simulink library "MBDS_Applications"  (R2018b)
settings: Solver=ode45  StartTime=0.0  StopTime=10.0  RelTol=1e-3
undefined symbols (not defined in the file or in its folder): Ts
libraries: KIBES_Signal x297, simulink x7
(part 1 of 6)
Description:
  | MBDS project library for Application models
settings Model: Creator=uid60719  LastModifiedBy=uidf0608
settings DataIOCC: LimitDataPoints=on  SaveFormat=Array  SignalLoggingSaveFormat=ModelDataLogs
settings OptimizationCC: BlockReduction=off  BooleanDataType=off  ExpressionDepthLimit=2147483647  LifeSpan=inf
settings DebuggingCC: SaveWithParameterizedLinksMsg=none  UnderspecifiedInitializationDetection=Classic  MergeDetectMultiDrivingBlocksExec=none  SignalResolutionControl=TryResolveAllWithWarning  MultiTaskCondExecSysMsg=none  FcnCallInpInsideContextMsg=warning  AllowSymbolicDim=off  StateNameClashWarn=warning  SFUnexpectedBacktrackingDiag=warning  SFNoUnconditionalDefaultTransitionDiag=warning  SFExecutionAtInitializationDiag=none
settings HardwareCC: ProdBitPerPointer=32  ProdBitPerSizeT=32  ProdBitPerPtrDiffT=32  ProdLargestAtomicFloat=None  ProdIntDivRoundTo=Undefined  ProdEndianess=Unspecified  ProdWordSize=32  ProdHWDeviceType=32-bit Generic  TargetUnknown=on
settings ModelReferenceCC: PropagateSignalLabelsOutOfModel=off
settings SFSimCC: SimUseLocalCustomCode=off
settings RTWCC: RTWUseLocalCustomCode=off
settings CodeAppCC: StateflowObjectComments=on
settings GRTTargetCC: TargetLangStandard=C89/C90 (ANSI)  GeneratePreprocessorConditionals=Disable all  CombineOutputUpdateFcns=off  GRTInterface=on
settings ConfigComp: CovMetricSettings=dw  CovHtmlReporting=on  CovSaveCumulativeToWorkspaceVar=on  CovSaveSingleToWorkspaceVar=on  CovExternalEMLEnable=off  CovSFcnEnable=off

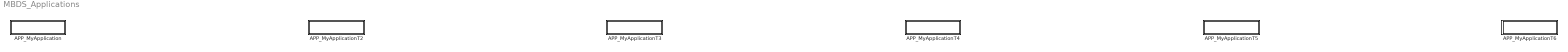
== system MBDS_Applications ==
  APP_MyApplication : Subsystem  mask(APP_MyApplication){MBDS_ElementType=Application, MBDS_WorkStatus=In Work, MBDS_LastModified=2021-02-03-13:46:18}
      mask prompts: MBDS_ElementType "MBDS element type:"; MBDS_WorkStatus "Work status:"; MBDS_LastModified "Last modified:"
      mask help: MBDS Application APP_MyApplication
      settings: CopyFcn=|
      | if(~strcmpi(GetElementType(bdroot(gcs)), 'System'))
      | RemoveBlockMsg(gcb, 'Application blocks can be used in system design models only. The added block instance will be removed from your model to avoid errors.');
      | end
      mask Help: eval(['open([workdir(''help_dir:''),''\MBDS_ProjectLibrary.html''])'])
      mask Display: disp('V 1.115')
  APP_MyApplicationT2 : Subsystem  Description=MyApplicationT2  mask(APP_MyApplicationT2){MBDS_ElementType=Application, MBDS_WorkStatus=In Work, MBDS_LastModified=2021-02-03-13:46:32}
      mask prompts: MBDS_ElementType "MBDS element type:"; MBDS_WorkStatus "Work status:"; MBDS_LastModified "Last modified:"
      mask help: MyApplicationT2
      settings: CopyFcn=|
      | if(~strcmpi(GetElementType(bdroot(gcs)), 'System'))
      | RemoveBlockMsg(gcb, 'Application blocks can be used in system design models only. The added block instance will be removed from your model to avoid errors.');
      | end
      mask Help: eval(['open([workdir(''help_dir:''),''\MBDS_ProjectLibrary.html''])'])
      mask Display: disp('V 1.5')
  APP_MyApplicationT3 : Subsystem  Description=MyApplicationT3  mask(APP_MyApplicationT3){MBDS_ElementType=Application, MBDS_WorkStatus=In Work, MBDS_LastModified=2021-02-03-13:46:39}
      mask prompts: MBDS_ElementType "MBDS element type:"; MBDS_WorkStatus "Work status:"; MBDS_LastModified "Last modified:"
      mask help: MyApplicationT3
      settings: CopyFcn=|
      | if(~strcmpi(GetElementType(bdroot(gcs)), 'System'))
      | RemoveBlockMsg(gcb, 'Application blocks can be used in system design models only. The added block instance will be removed from your model to avoid errors.');
      | end
      mask Help: eval(['open([workdir(''help_dir:''),''\MBDS_ProjectLibrary.html''])'])
      mask Display: disp('V 1.3')
  APP_MyApplicationT4 : Subsystem  Description=MyApplicationT4  mask(APP_MyApplicationT4){MBDS_ElementType=Application, MBDS_WorkStatus=In Work, MBDS_LastModified=2021-02-03-13:46:48}
      mask prompts: MBDS_ElementType "MBDS element type:"; MBDS_WorkStatus "Work status:"; MBDS_LastModified "Last modified:"
      mask help: MyApplicationT4
      settings: CopyFcn=|
      | if(~strcmpi(GetElementType(bdroot(gcs)), 'System'))
      | RemoveBlockMsg(gcb, 'Application blocks can be used in system design models only. The added block instance will be removed from your model to avoid errors.');
      | end
      mask Help: eval(['open([workdir(''help_dir:''),''\MBDS_ProjectLibrary.html''])'])
      mask Display: disp('V 1.11')
  APP_MyApplicationT5 : Subsystem  Description=MyApplicationT5  mask(APP_MyApplicationT5){MBDS_ElementType=Application, MBDS_WorkStatus=In Work, MBDS_LastModified=2021-02-03-13:46:56}
      mask prompts: MBDS_ElementType "MBDS element type:"; MBDS_WorkStatus "Work status:"; MBDS_LastModified "Last modified:"
      mask help: MyApplicationT5
      settings: CopyFcn=|
      | if(~strcmpi(GetElementType(bdroot(gcs)), 'System'))
      | RemoveBlockMsg(gcb, 'Application blocks can be used in system design models only. The added block instance will be removed from your model to avoid errors.');
      | end
      mask Help: eval(['open([workdir(''help_dir:''),''\MBDS_ProjectLibrary.html''])'])
      mask Display: disp('V 1.9')
  APP_MyApplicationT6 : Subsystem  Description=MyApplicationT6  mask(APP_MyApplicationT6){MBDS_ElementType=Application, MBDS_WorkStatus=In Work, MBDS_LastModified=2021-02-03-13:47:04}
      mask prompts: MBDS_ElementType "MBDS element type:"; MBDS_WorkStatus "Work status:"; MBDS_LastModified "Last modified:"
      mask help: MyApplicationT6
      settings: CopyFcn=|
      | if(~strcmpi(GetElementType(bdroot(gcs)), 'System'))
      | RemoveBlockMsg(gcb, 'Application blocks can be used in system design models only. The added block instance will be removed from your model to avoid errors.');
      | end
      mask Help: eval(['open([workdir(''help_dir:''),''\MBDS_ProjectLibrary.html''])'])
      mask Display: disp('V 1.5')

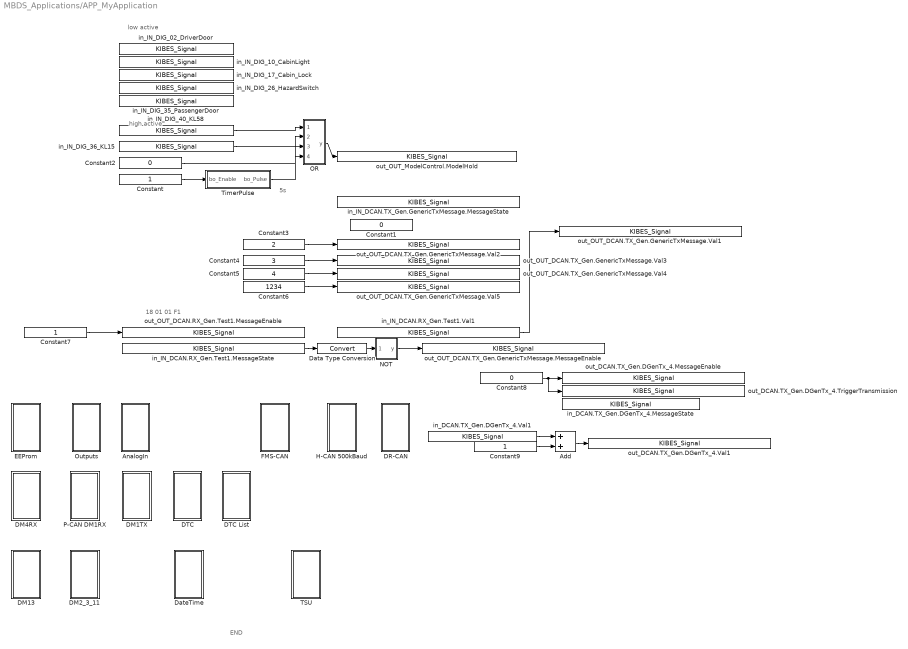
== system MBDS_Applications/APP_MyApplication ==
  note: low active
  note: 5s
  note: high active
  note: 18 01 01 F1
  note: END
  Add : Sum  InitFcn=|  OutDataTypeStr=Inherit: Inherit via back propagation  SaturateOnIntegerOverflow=on
      | if(exist('MBDS_BlockCallback', 'file'))
      |    MBDS_BlockCallback('Update', gcb);  
      | end
      settings: AttributesFormatString=Saturate: %<SaturateOnIntegerOverflow>
  AnalogIn : Subsystem
  Constant : Constant  InitFcn=|  OutDataTypeStr=boolean
      | if(exist('MBDS_BlockCallback', 'file'))
      |    MBDS_BlockCallback('Update', gcb);  
      | end
  Constant1 : Constant  InitFcn=|  Value=0  OutDataTypeStr=boolean
      | if(exist('MBDS_BlockCallback', 'file'))
      |    MBDS_BlockCallback('Update', gcb);  
      | end
  Constant2 : Constant  InitFcn=|  Value=0  OutDataTypeStr=boolean
      | if(exist('MBDS_BlockCallback', 'file'))
      |    MBDS_BlockCallback('Update', gcb);  
      | end
  Constant3 : Constant  InitFcn=|  Value=2  OutDataTypeStr=uint8
      | if(exist('MBDS_BlockCallback', 'file'))
      |    MBDS_BlockCallback('Update', gcb);  
      | end
  Constant4 : Constant  InitFcn=|  Value=3  OutDataTypeStr=uint8
      | if(exist('MBDS_BlockCallback', 'file'))
      |    MBDS_BlockCallback('Update', gcb);  
      | end
  Constant5 : Constant  InitFcn=|  Value=4  OutDataTypeStr=uint8
      | if(exist('MBDS_BlockCallback', 'file'))
      |    MBDS_BlockCallback('Update', gcb);  
      | end
  Constant6 : Constant  InitFcn=|  Value=1234  OutDataTypeStr=uint32
      | if(exist('MBDS_BlockCallback', 'file'))
      |    MBDS_BlockCallback('Update', gcb);  
      | end
  Constant7 : Constant  InitFcn=|  OutDataTypeStr=boolean
      | if(exist('MBDS_BlockCallback', 'file'))
      |    MBDS_BlockCallback('Update', gcb);  
      | end
  Constant8 : Constant  InitFcn=|  Value=0  OutDataTypeStr=boolean
      | if(exist('MBDS_BlockCallback', 'file'))
      |    MBDS_BlockCallback('Update', gcb);  
      | end
  Constant9 : Constant  InitFcn=|  OutDataTypeStr=uint32
      | if(exist('MBDS_BlockCallback', 'file'))
      |    MBDS_BlockCallback('Update', gcb);  
      | end
  DM13 : Subsystem
  DM1TX : Subsystem
  DM2_3_11 : Subsystem
  DM4RX : Subsystem
  DR-CAN : Subsystem
  DTC : Subsystem
  DTC List : Subsystem
  Data Type Conversion : DataTypeConversion  InitFcn=|  SaturateOnIntegerOverflow=on
      | try
      |    MBDS_BlockCallback('Update', gcb);
      | end
      settings: AttributesFormatString=Saturate: %<SaturateOnIntegerOverflow>
  DateTime : Subsystem
  EEProm : Subsystem
  FMS-CAN : Subsystem
  H-CAN 500kBaud : Subsystem
  NOT : Subsystem  InitFcn=|  mask(NOT){MBDS_LibraryBlock=on, BitwiseMode=off, Inputs=1, UseBitMask=off, BitMask='A1', OutDataTypeStr=Inherit: Inherit via back propagation, MBDS_BlockVersion=07.21.05}
      | if(exist('MBDS_BlockCallback', 'file'))
      |    MBDS_BlockCallback('Update', gcb);
      | end
      mask prompts: MBDS_LibraryBlock "MBDS library block"; BitwiseMode "Use 'bitwise' mode"; Inputs "Number of input ports:"; UseBitMask "Use bit mask"; BitMask "Bit mask:"; OutDataTypeStr "Output data type:"; MBDS_BlockVersion "Version:"
      mask help: Logical or bitwise NOT operator. The input value is inverted. In bitwise mode all bits of the input signal are inverted.
      mask init:
      | if(exist('MBDS_BlockCallback', 'file'))
      |    MBDS_BlockCallback('Init', gcb);
      | else
      |    % Disable all mask parameters
      |    MaskEnables = get_param(gcb, 'MaskEnables');
      |    for k = [1:length(MaskEnables)]
      |       MaskEnables{k} = 'off';
      |    end
      |    if(~isequal(MaskEnables, get_param(gcb, 'MaskEnables')))
      |       set_param(gcb, 'MaskEnables', MaskEnables);
      |    end
      | end
      mask Help: eval(['open([workdir(''library_dir:''),''\Blockset\help\'',get_param(gcb,''MaskType''),''.html''])'])
      mask Callback BitwiseMode:
      | if(exist('MBDS_BlockCallback', 'file'))
      |    MBDS_BlockCallback('BitwiseMode', gcb);
      | end
      mask TypeOptions OutDataTypeStr: Inherit: Inherit via back propagation | int8 | uint8 | int16 | uint16 | int32 | uint32 | boolean
      mask Callback OutDataTypeStr:
      | % Adopt Value
      | if(exist('MBDS_BlockCallback', 'file'))
      |    MBDS_BlockCallback('OutDataTypeStr', gcb);
      | end
      mask DialogControl ParameterTabVar0 Prompt: Main
      mask DialogControl ParameterTabVar01 Prompt: Signal Attributes
      mask DialogControl ParameterTabVar012 Prompt: Version
      mask Display:
      | % Show icon or block text
      | disp('NOT')
  OR : Subsystem  InitFcn=|  mask(OR){MBDS_LibraryBlock=on, BitwiseMode=off, Inputs=4, UseBitMask=off, BitMask='A1', OutDataTypeStr=Inherit: Inherit via back propagation, MBDS_BlockVersion=07.21.05}
      | if(exist('MBDS_BlockCallback', 'file'))
      |    MBDS_BlockCallback('Update', gcb);
      | end
      mask prompts: MBDS_LibraryBlock "MBDS library block"; BitwiseMode "Use 'bitwise' mode"; Inputs "Number of input ports:"; UseBitMask "Use bit mask"; BitMask "Bit mask:"; OutDataTypeStr "Output data type:"; MBDS_BlockVersion "Version:"
      mask help: Logical or bitwise OR operator. For multiple inputs, operators are applied across the inputs. For a single input, operators are applied across the input vector. In bitwise mode a bit mask can be applied onto single input signals.
      mask init: same as MBDS_Applications/APP_MyApplication/NOT
      mask Help: eval(['open([workdir(''library_dir:''),''\Blockset\help\'',get_param(gcb,''MaskType''),''.html''])'])
      mask Callback BitwiseMode:
      | if(exist('MBDS_BlockCallback', 'file'))
      |    MBDS_BlockCallback('BitwiseMode', gcb);
      | end
      mask Callback Inputs:
      | if(exist('MBDS_BlockCallback', 'file'))
      |    MBDS_BlockCallback('Inputs', gcb);
      | end
      mask Callback UseBitMask:
      | if(exist('MBDS_BlockCallback', 'file'))
      |    MBDS_BlockCallback('UseBitMask', gcb);
      | end
      mask Callback BitMask:
      | if(exist('MBDS_BlockCallback', 'file'))
      |    MBDS_BlockCallback('BitMask', gcb);
      | end
      mask TypeOptions OutDataTypeStr: Inherit: Inherit via back propagation | int8 | uint8 | int16 | uint16 | int32 | uint32 | boolean
      mask Callback OutDataTypeStr:
      | % Adopt Value
      | if(exist('MBDS_BlockCallback', 'file'))
      |    MBDS_BlockCallback('OutDataTypeStr', gcb);
      | end
      mask DialogControl ParameterTabVar0 Prompt: Main
      mask DialogControl ParameterTabVar01 Prompt: Signal Attributes
      mask DialogControl ParameterTabVar012 Prompt: Version
      mask Display:
      | % Show icon or block text
      | if(UseBitMask)
      |    if(isnumeric(BitMask))
      |       BitMaskString = ['0x',dec2hex(floor(BitMask))];
      |    elseif(ischar(BitMask))
      |       BitMaskString = ['0x',upper(BitMask)];
      |    else
      |       BitMaskString = '???';
      |    end
      |    disp(sprintf(['OR\n', BitMaskString]))
      | else
      |    disp('OR')
      | end
  Outputs : Subsystem
  P-CAN DM1RX : Subsystem
  TSU : Subsystem
  TimerPulse : Subsystem
  in_DCAN.TX_Gen.DGenTx_4.MessageState : KIBES_Signal/KIBES_Signal  MBDS_LibraryBlock=on  DatabaseKey=271  SignalName=DCAN.TX_Gen.DGenTx_4.MessageState  SymbolName=DCAN_TX_Gen_DGenTx_4_MessageState_000271  DataType=uint16  Init=0  Slope=1  Bias=0  DataSize=1  fpDataType=uint16  BlockIOType=Inport  DeviceType=0
  in_DCAN.TX_Gen.DGenTx_4.Val1 : KIBES_Signal/KIBES_Signal  MBDS_LibraryBlock=on  DatabaseKey=272  SignalName=DCAN.TX_Gen.DGenTx_4.Val1  SymbolName=DCAN_TX_Gen_DGenTx_4_Val1_000272  DataType=uint32  Init=0  Slope=1  Bias=0  DataSize=1  fpDataType=uint32  BlockIOType=Inport  DeviceType=0
  in_IN_DCAN.RX_Gen.Test1.MessageState : KIBES_Signal/KIBES_Signal  MBDS_LibraryBlock=on  DatabaseKey=10  SignalName=IN_DCAN.RX_Gen.Test1.MessageState  SymbolName=IN_DCAN_RX_Gen_Test1_MessageState_000010  DataType=uint16  Init=0  Slope=1  Bias=0  DataSize=1  fpDataType=uint16  BlockIOType=Inport  DeviceType=0
  in_IN_DCAN.RX_Gen.Test1.Val1 : KIBES_Signal/KIBES_Signal  MBDS_LibraryBlock=on  DatabaseKey=11  SignalName=IN_DCAN.RX_Gen.Test1.Val1  SymbolName=IN_DCAN_RX_Gen_Test1_Val1_000011  DataType=uint8  Init=0  Slope=1  Bias=0  DataSize=1  fpDataType=uint8  BlockIOType=Inport  DeviceType=0
  in_IN_DCAN.TX_Gen.GenericTxMessage.MessageState : KIBES_Signal/KIBES_Signal  MBDS_LibraryBlock=on  DatabaseKey=3  SignalName=IN_DCAN.TX_Gen.GenericTxMessage.MessageState  SymbolName=IN_DCAN_TX_Gen_GenericTxMessage_MessageState_000003  DataType=uint16  Init=0  Slope=1  Bias=0  DataSize=1  fpDataType=uint16  BlockIOType=Inport  DeviceType=0
  in_IN_DIG_02_DriverDoor : KIBES_Signal/KIBES_Signal  MBDS_LibraryBlock=on  DatabaseKey=215  SignalName=IN_DIG_02_DriverDoor  SymbolName=IN_DIG_02_DriverDoor_000215  DataType=boolean  Init=0  Slope=1  Bias=0  DataSize=1  fpDataType=boolean  BlockIOType=Inport  DeviceType=0
  in_IN_DIG_10_CabinLight : KIBES_Signal/KIBES_Signal  MBDS_LibraryBlock=on  DatabaseKey=213  SignalName=IN_DIG_10_CabinLight  SymbolName=IN_DIG_10_CabinLight_000213  DataType=boolean  Init=0  Slope=1  Bias=0  DataSize=1  fpDataType=boolean  BlockIOType=Inport  DeviceType=0
  in_IN_DIG_17_Cabin_Lock : KIBES_Signal/KIBES_Signal  MBDS_LibraryBlock=on  DatabaseKey=211  SignalName=IN_DIG_17_Cabin_Lock  SymbolName=IN_DIG_17_Cabin_Lock_000211  DataType=boolean  Init=0  Slope=1  Bias=0  DataSize=1  fpDataType=boolean  BlockIOType=Inport  DeviceType=0
  in_IN_DIG_26_HazardSwitch : KIBES_Signal/KIBES_Signal  MBDS_LibraryBlock=on  DatabaseKey=212  SignalName=IN_DIG_26_HazardSwitch  SymbolName=IN_DIG_26_HazardSwitch_000212  DataType=boolean  Init=0  Slope=1  Bias=0  DataSize=1  fpDataType=boolean  BlockIOType=Inport  DeviceType=0
  in_IN_DIG_35_PassengerDoor : KIBES_Signal/KIBES_Signal  MBDS_LibraryBlock=on  DatabaseKey=214  SignalName=IN_DIG_35_PassengerDoor  SymbolName=IN_DIG_35_PassengerDoor_000214  DataType=boolean  Init=0  Slope=1  Bias=0  DataSize=1  fpDataType=boolean  BlockIOType=Inport  DeviceType=0
  in_IN_DIG_36_KL15 : KIBES_Signal/KIBES_Signal  MBDS_LibraryBlock=on  DatabaseKey=216  SignalName=IN_DIG_36_KL15  SymbolName=IN_DIG_36_KL15_000216  DataType=boolean  Init=0  Slope=1  Bias=0  DataSize=1  fpDataType=boolean  BlockIOType=Inport  DeviceType=0
  in_IN_DIG_40_KL58 : KIBES_Signal/KIBES_Signal  MBDS_LibraryBlock=on  DatabaseKey=210  SignalName=IN_DIG_40_KL58  SymbolName=IN_DIG_40_KL58_000210  DataType=boolean  Init=0  Slope=1  Bias=0  DataSize=1  fpDataType=boolean  BlockIOType=Inport  DeviceType=0
  out_DCAN.TX_Gen.DGenTx_4.MessageEnable : KIBES_Signal/KIBES_Signal  MBDS_LibraryBlock=on  DatabaseKey=270  SignalName=DCAN.TX_Gen.DGenTx_4.MessageEnable  SymbolName=DCAN_TX_Gen_DGenTx_4_MessageEnable_000270  DataType=boolean  Init=0  Slope=1  Bias=0  DataSize=1  fpDataType=boolean  BlockIOType=Outport  DeviceType=0
  out_DCAN.TX_Gen.DGenTx_4.TriggerTransmission : KIBES_Signal/KIBES_Signal  MBDS_LibraryBlock=on  DatabaseKey=273  SignalName=DCAN.TX_Gen.DGenTx_4.TriggerTransmission  SymbolName=DCAN_TX_Gen_DGenTx_4_TriggerTransmission_000273  DataType=boolean  Init=0  Slope=1  Bias=0  DataSize=1  fpDataType=boolean  BlockIOType=Outport  DeviceType=0
  out_DCAN.TX_Gen.DGenTx_4.Val1 : KIBES_Signal/KIBES_Signal  MBDS_LibraryBlock=on  DatabaseKey=272  SignalName=DCAN.TX_Gen.DGenTx_4.Val1  SymbolName=DCAN_TX_Gen_DGenTx_4_Val1_000272  DataType=uint32  Init=0  Slope=1  Bias=0  DataSize=1  fpDataType=uint32  BlockIOType=Outport  DeviceType=0
  out_OUT_DCAN.RX_Gen.Test1.MessageEnable : KIBES_Signal/KIBES_Signal  MBDS_LibraryBlock=on  DatabaseKey=9  SignalName=OUT_DCAN.RX_Gen.Test1.MessageEnable  SymbolName=OUT_DCAN_RX_Gen_Test1_MessageEnable_000009  DataType=boolean  Init=0  Slope=1  Bias=0  DataSize=1  fpDataType=boolean  BlockIOType=Outport  DeviceType=0
  out_OUT_DCAN.TX_Gen.GenericTxMessage.MessageEnable : KIBES_Signal/KIBES_Signal  MBDS_LibraryBlock=on  DatabaseKey=2  SignalName=OUT_DCAN.TX_Gen.GenericTxMessage.MessageEnable  SymbolName=OUT_DCAN_TX_Gen_GenericTxMessage_MessageEnable_000002  DataType=boolean  Init=0  Slope=1  Bias=0  DataSize=1  fpDataType=boolean  BlockIOType=Outport  DeviceType=0
  out_OUT_DCAN.TX_Gen.GenericTxMessage.Val1 : KIBES_Signal/KIBES_Signal  MBDS_LibraryBlock=on  DatabaseKey=4  SignalName=OUT_DCAN.TX_Gen.GenericTxMessage.Val1  SymbolName=OUT_DCAN_TX_Gen_GenericTxMessage_Val1_000004  DataType=uint8  Init=0  Slope=1  Bias=0  DataSize=1  fpDataType=uint8  BlockIOType=Outport  DeviceType=0
  out_OUT_DCAN.TX_Gen.GenericTxMessage.Val2 : KIBES_Signal/KIBES_Signal  MBDS_LibraryBlock=on  DatabaseKey=5  SignalName=OUT_DCAN.TX_Gen.GenericTxMessage.Val2  SymbolName=OUT_DCAN_TX_Gen_GenericTxMessage_Val2_000005  DataType=uint8  Init=0  Slope=1  Bias=0  DataSize=1  fpDataType=uint8  BlockIOType=Outport  DeviceType=0
  out_OUT_DCAN.TX_Gen.GenericTxMessage.Val3 : KIBES_Signal/KIBES_Signal  MBDS_LibraryBlock=on  DatabaseKey=6  SignalName=OUT_DCAN.TX_Gen.GenericTxMessage.Val3  SymbolName=OUT_DCAN_TX_Gen_GenericTxMessage_Val3_000006  DataType=uint8  Init=0  Slope=1  Bias=0  DataSize=1  fpDataType=uint8  BlockIOType=Outport  DeviceType=0
  out_OUT_DCAN.TX_Gen.GenericTxMessage.Val4 : KIBES_Signal/KIBES_Signal  MBDS_LibraryBlock=on  DatabaseKey=7  SignalName=OUT_DCAN.TX_Gen.GenericTxMessage.Val4  SymbolName=OUT_DCAN_TX_Gen_GenericTxMessage_Val4_000007  DataType=uint8  Init=0  Slope=1  Bias=0  DataSize=1  fpDataType=uint8  BlockIOType=Outport  DeviceType=0
  out_OUT_DCAN.TX_Gen.GenericTxMessage.Val5 : KIBES_Signal/KIBES_Signal  MBDS_LibraryBlock=on  DatabaseKey=8  SignalName=OUT_DCAN.TX_Gen.GenericTxMessage.Val5  SymbolName=OUT_DCAN_TX_Gen_GenericTxMessage_Val5_000008  DataType=uint32  Init=0  Slope=1  Bias=0  DataSize=1  fpDataType=uint32  BlockIOType=Outport  DeviceType=0
  out_OUT_ModelControl.ModelHold : KIBES_Signal/KIBES_Signal  MBDS_LibraryBlock=on  DatabaseKey=1  SignalName=OUT_ModelControl.ModelHold  SymbolName=OUT_ModelControl_ModelHold_000001  DataType=boolean  Init=0  Slope=1  Bias=0  DataSize=1  fpDataType=boolean  BlockIOType=Outport  DeviceType=0
  wires:
  TimerPulse/1(bo_Pulse) -> OR/4(u4)
  Constant2/1 -> OR/3(u3)
  Add/1 -> out_DCAN.TX_Gen.DGenTx_4.Val1/1
  Constant3/1 -> out_OUT_DCAN.TX_Gen.GenericTxMessage.Val2/1
  Constant8/1 -> out_DCAN.TX_Gen.DGenTx_4.MessageEnable/1, out_DCAN.TX_Gen.DGenTx_4.TriggerTransmission/1
  Constant9/1 -> Add/2
  in_DCAN.TX_Gen.DGenTx_4.Val1/1 -> Add/1
  NOT/1(y) -> out_OUT_DCAN.TX_Gen.GenericTxMessage.MessageEnable/1
  Data Type Conversion/1 -> NOT/1(u1)
  in_IN_DCAN.RX_Gen.Test1.MessageState/1 -> Data Type Conversion/1
  in_IN_DIG_36_KL15/1 -> OR/2(u2)
  OR/1(y) -> out_OUT_ModelControl.ModelHold/1
  in_IN_DIG_40_KL58/1 -> OR/1(u1)
  Constant/1 -> TimerPulse/1(bo_Enable)
  Constant7/1 -> out_OUT_DCAN.RX_Gen.Test1.MessageEnable/1
  Constant6/1 -> out_OUT_DCAN.TX_Gen.GenericTxMessage.Val5/1
  Constant5/1 -> out_OUT_DCAN.TX_Gen.GenericTxMessage.Val4/1
  Constant4/1 -> out_OUT_DCAN.TX_Gen.GenericTxMessage.Val3/1
  in_IN_DCAN.RX_Gen.Test1.Val1/1 -> out_OUT_DCAN.TX_Gen.GenericTxMessage.Val1/1

== system MBDS_Applications/APP_MyApplicationT2 ==
  in_IN_DigitalInputs.IN_DIG_01 : KIBES_Signal/KIBES_Signal  MBDS_LibraryBlock=on  DatabaseKey=73  SignalName=IN_DigitalInputs.IN_DIG_01  SymbolName=IN_DigitalInputs_IN_DIG_01_000073  DataType=boolean  Init=0  Slope=1  Bias=0  DataSize=1  fpDataType=boolean  BlockIOType=Inport  DeviceType=0

== system MBDS_Applications/APP_MyApplicationT3 ==
  in_IN_DigitalInputs.IN_DIG_01 : KIBES_Signal/KIBES_Signal  MBDS_LibraryBlock=on  DatabaseKey=73  SignalName=IN_DigitalInputs.IN_DIG_01  SymbolName=IN_DigitalInputs_IN_DIG_01_000073  DataType=boolean  Init=0  Slope=1  Bias=0  DataSize=1  fpDataType=boolean  BlockIOType=Inport  DeviceType=0

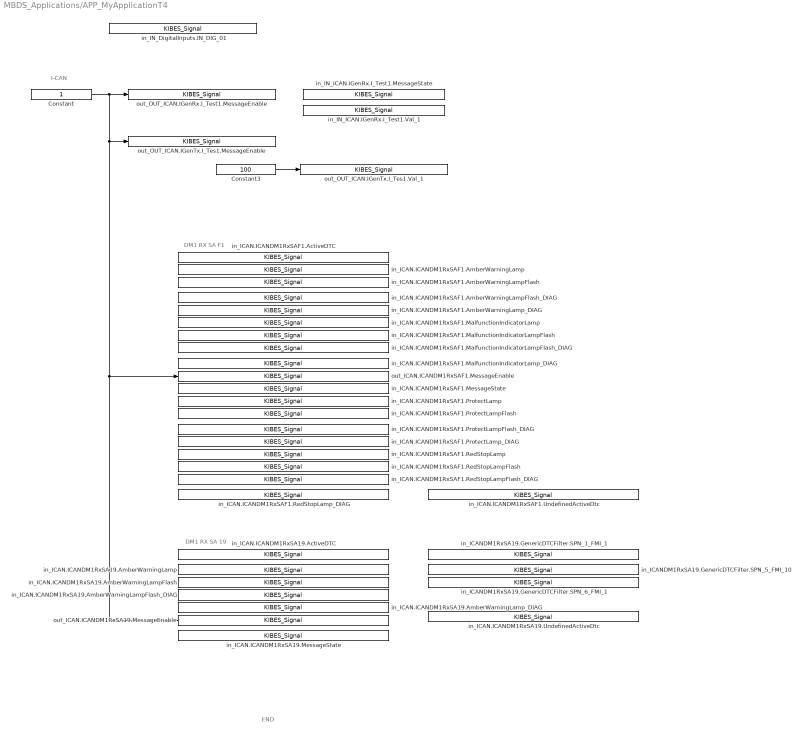
== system MBDS_Applications/APP_MyApplicationT4 ==
  note: I-CAN
  note: DM1 RX SA F1
  note: END
  note: DM1 RX SA 19
  Constant : Constant  InitFcn=|  OutDataTypeStr=boolean
      | if(exist('MBDS_BlockCallback', 'file'))
      |    MBDS_BlockCallback('Update', gcb);  
      | end
  Constant3 : Constant  InitFcn=|  Value=100  OutDataTypeStr=uint8
      | if(exist('MBDS_BlockCallback', 'file'))
      |    MBDS_BlockCallback('Update', gcb);  
      | end
  in_ICAN.ICANDM1RxSA19.ActiveDTC : KIBES_Signal/KIBES_Signal  MBDS_LibraryBlock=on  DatabaseKey=149  SignalName=ICAN.ICANDM1RxSA19.ActiveDTC  SymbolName=ICAN_ICANDM1RxSA19_ActiveDTC_000149  DataType=boolean  Init=0  Slope=1  Bias=0  DataSize=1  fpDataType=boolean  BlockIOType=Inport  DeviceType=0
  in_ICAN.ICANDM1RxSA19.AmberWarningLamp : KIBES_Signal/KIBES_Signal  MBDS_LibraryBlock=on  DatabaseKey=150  SignalName=ICAN.ICANDM1RxSA19.AmberWarningLamp  SymbolName=ICAN_ICANDM1RxSA19_AmberWarningLamp_000150  DataType=boolean  Init=0  Slope=1  Bias=0  DataSize=1  fpDataType=boolean  BlockIOType=Inport  DeviceType=0
  in_ICAN.ICANDM1RxSA19.AmberWarningLampFlash : KIBES_Signal/KIBES_Signal  MBDS_LibraryBlock=on  DatabaseKey=151  SignalName=ICAN.ICANDM1RxSA19.AmberWarningLampFlash  SymbolName=ICAN_ICANDM1RxSA19_AmberWarningLampFlash_000151  DataType=uint8  Init=0  Slope=1  Bias=0  DataSize=1  fpDataType=uint8  BlockIOType=Inport  DeviceType=0
  in_ICAN.ICANDM1RxSA19.AmberWarningLampFlash_DIAG : KIBES_Signal/KIBES_Signal  MBDS_LibraryBlock=on  DatabaseKey=152  SignalName=ICAN.ICANDM1RxSA19.AmberWarningLampFlash_DIAG  SymbolName=ICAN_ICANDM1RxSA19_AmberWarningLampFlash_DIAG_000152  DataType=uint16  Init=1  Slope=1  Bias=0  DataSize=1  fpDataType=uint16  BlockIOType=Inport  DeviceType=0
  in_ICAN.ICANDM1RxSA19.AmberWarningLamp_DIAG : KIBES_Signal/KIBES_Signal  MBDS_LibraryBlock=on  DatabaseKey=153  SignalName=ICAN.ICANDM1RxSA19.AmberWarningLamp_DIAG  SymbolName=ICAN_ICANDM1RxSA19_AmberWarningLamp_DIAG_000153  DataType=uint16  Init=1  Slope=1  Bias=0  DataSize=1  fpDataType=uint16  BlockIOType=Inport  DeviceType=0
  in_ICAN.ICANDM1RxSA19.MessageState : KIBES_Signal/KIBES_Signal  MBDS_LibraryBlock=on  DatabaseKey=155  SignalName=ICAN.ICANDM1RxSA19.MessageState  SymbolName=ICAN_ICANDM1RxSA19_MessageState_000155  DataType=uint16  Init=0  Slope=1  Bias=0  DataSize=1  fpDataType=uint16  BlockIOType=Inport  DeviceType=0
  in_ICAN.ICANDM1RxSA19.UndefinedActiveDtc : KIBES_Signal/KIBES_Signal  MBDS_LibraryBlock=on  DatabaseKey=401  SignalName=ICAN.ICANDM1RxSA19.UndefinedActiveDtc  SymbolName=ICAN_ICANDM1RxSA19_UndefinedActiveDtc_000401  DataType=boolean  Init=0  Slope=1  Bias=0  DataSize=1  fpDataType=boolean  BlockIOType=Inport  DeviceType=0
  in_ICAN.ICANDM1RxSAF1.ActiveDTC : KIBES_Signal/KIBES_Signal  MBDS_LibraryBlock=on  DatabaseKey=129  SignalName=ICAN.ICANDM1RxSAF1.ActiveDTC  SymbolName=ICAN_ICANDM1RxSAF1_ActiveDTC_000129  DataType=boolean  Init=0  Slope=1  Bias=0  DataSize=1  fpDataType=boolean  BlockIOType=Inport  DeviceType=0
  in_ICAN.ICANDM1RxSAF1.AmberWarningLamp : KIBES_Signal/KIBES_Signal  MBDS_LibraryBlock=on  DatabaseKey=130  SignalName=ICAN.ICANDM1RxSAF1.AmberWarningLamp  SymbolName=ICAN_ICANDM1RxSAF1_AmberWarningLamp_000130  DataType=boolean  Init=0  Slope=1  Bias=0  DataSize=1  fpDataType=boolean  BlockIOType=Inport  DeviceType=0
  in_ICAN.ICANDM1RxSAF1.AmberWarningLampFlash : KIBES_Signal/KIBES_Signal  MBDS_LibraryBlock=on  DatabaseKey=131  SignalName=ICAN.ICANDM1RxSAF1.AmberWarningLampFlash  SymbolName=ICAN_ICANDM1RxSAF1_AmberWarningLampFlash_000131  DataType=uint8  Init=0  Slope=1  Bias=0  DataSize=1  fpDataType=uint8  BlockIOType=Inport  DeviceType=0
  in_ICAN.ICANDM1RxSAF1.AmberWarningLampFlash_DIAG : KIBES_Signal/KIBES_Signal  MBDS_LibraryBlock=on  DatabaseKey=132  SignalName=ICAN.ICANDM1RxSAF1.AmberWarningLampFlash_DIAG  SymbolName=ICAN_ICANDM1RxSAF1_AmberWarningLampFlash_DIAG_000132  DataType=uint16  Init=1  Slope=1  Bias=0  DataSize=1  fpDataType=uint16  BlockIOType=Inport  DeviceType=0
  in_ICAN.ICANDM1RxSAF1.AmberWarningLamp_DIAG : KIBES_Signal/KIBES_Signal  MBDS_LibraryBlock=on  DatabaseKey=133  SignalName=ICAN.ICANDM1RxSAF1.AmberWarningLamp_DIAG  SymbolName=ICAN_ICANDM1RxSAF1_AmberWarningLamp_DIAG_000133  DataType=uint16  Init=1  Slope=1  Bias=0  DataSize=1  fpDataType=uint16  BlockIOType=Inport  DeviceType=0
  in_ICAN.ICANDM1RxSAF1.MalfunctionIndicatorLamp : KIBES_Signal/KIBES_Signal  MBDS_LibraryBlock=on  DatabaseKey=134  SignalName=ICAN.ICANDM1RxSAF1.MalfunctionIndicatorLamp  SymbolName=ICAN_ICANDM1RxSAF1_MalfunctionIndicatorLamp_000134  DataType=boolean  Init=0  Slope=1  Bias=0  DataSize=1  fpDataType=boolean  BlockIOType=Inport  DeviceType=0
  in_ICAN.ICANDM1RxSAF1.MalfunctionIndicatorLampFlash : KIBES_Signal/KIBES_Signal  MBDS_LibraryBlock=on  DatabaseKey=135  SignalName=ICAN.ICANDM1RxSAF1.MalfunctionIndicatorLampFlash  SymbolName=ICAN_ICANDM1RxSAF1_MalfunctionIndicatorLampFlash_000135  DataType=uint8  Init=0  Slope=1  Bias=0  DataSize=1  fpDataType=uint8  BlockIOType=Inport  DeviceType=0
  in_ICAN.ICANDM1RxSAF1.MalfunctionIndicatorLampFlash_DIAG : KIBES_Signal/KIBES_Signal  MBDS_LibraryBlock=on  DatabaseKey=136  SignalName=ICAN.ICANDM1RxSAF1.MalfunctionIndicatorLampFlash_DIAG  SymbolName=ICAN_ICANDM1RxSAF1_MalfunctionIndicatorLampFlash_DIAG_000136  DataType=uint16  Init=1  Slope=1  Bias=0  DataSize=1  fpDataType=uint16  BlockIOType=Inport  DeviceType=0
  in_ICAN.ICANDM1RxSAF1.MalfunctionIndicatorLamp_DIAG : KIBES_Signal/KIBES_Signal  MBDS_LibraryBlock=on  DatabaseKey=137  SignalName=ICAN.ICANDM1RxSAF1.MalfunctionIndicatorLamp_DIAG  SymbolName=ICAN_ICANDM1RxSAF1_MalfunctionIndicatorLamp_DIAG_000137  DataType=uint16  Init=1  Slope=1  Bias=0  DataSize=1  fpDataType=uint16  BlockIOType=Inport  DeviceType=0
  in_ICAN.ICANDM1RxSAF1.MessageState : KIBES_Signal/KIBES_Signal  MBDS_LibraryBlock=on  DatabaseKey=139  SignalName=ICAN.ICANDM1RxSAF1.MessageState  SymbolName=ICAN_ICANDM1RxSAF1_MessageState_000139  DataType=uint16  Init=0  Slope=1  Bias=0  DataSize=1  fpDataType=uint16  BlockIOType=Inport  DeviceType=0
  in_ICAN.ICANDM1RxSAF1.ProtectLamp : KIBES_Signal/KIBES_Signal  MBDS_LibraryBlock=on  DatabaseKey=140  SignalName=ICAN.ICANDM1RxSAF1.ProtectLamp  SymbolName=ICAN_ICANDM1RxSAF1_ProtectLamp_000140  DataType=boolean  Init=0  Slope=1  Bias=0  DataSize=1  fpDataType=boolean  BlockIOType=Inport  DeviceType=0
  in_ICAN.ICANDM1RxSAF1.ProtectLampFlash : KIBES_Signal/KIBES_Signal  MBDS_LibraryBlock=on  DatabaseKey=141  SignalName=ICAN.ICANDM1RxSAF1.ProtectLampFlash  SymbolName=ICAN_ICANDM1RxSAF1_ProtectLampFlash_000141  DataType=uint8  Init=0  Slope=1  Bias=0  DataSize=1  fpDataType=uint8  BlockIOType=Inport  DeviceType=0
  in_ICAN.ICANDM1RxSAF1.ProtectLampFlash_DIAG : KIBES_Signal/KIBES_Signal  MBDS_LibraryBlock=on  DatabaseKey=142  SignalName=ICAN.ICANDM1RxSAF1.ProtectLampFlash_DIAG  SymbolName=ICAN_ICANDM1RxSAF1_ProtectLampFlash_DIAG_000142  DataType=uint16  Init=1  Slope=1  Bias=0  DataSize=1  fpDataType=uint16  BlockIOType=Inport  DeviceType=0
  in_ICAN.ICANDM1RxSAF1.ProtectLamp_DIAG : KIBES_Signal/KIBES_Signal  MBDS_LibraryBlock=on  DatabaseKey=143  SignalName=ICAN.ICANDM1RxSAF1.ProtectLamp_DIAG  SymbolName=ICAN_ICANDM1RxSAF1_ProtectLamp_DIAG_000143  DataType=uint16  Init=1  Slope=1  Bias=0  DataSize=1  fpDataType=uint16  BlockIOType=Inport  DeviceType=0
  in_ICAN.ICANDM1RxSAF1.RedStopLamp : KIBES_Signal/KIBES_Signal  MBDS_LibraryBlock=on  DatabaseKey=144  SignalName=ICAN.ICANDM1RxSAF1.RedStopLamp  SymbolName=ICAN_ICANDM1RxSAF1_RedStopLamp_000144  DataType=boolean  Init=0  Slope=1  Bias=0  DataSize=1  fpDataType=boolean  BlockIOType=Inport  DeviceType=0
  in_ICAN.ICANDM1RxSAF1.RedStopLampFlash : KIBES_Signal/KIBES_Signal  MBDS_LibraryBlock=on  DatabaseKey=145  SignalName=ICAN.ICANDM1RxSAF1.RedStopLampFlash  SymbolName=ICAN_ICANDM1RxSAF1_RedStopLampFlash_000145  DataType=uint8  Init=0  Slope=1  Bias=0  DataSize=1  fpDataType=uint8  BlockIOType=Inport  DeviceType=0
  in_ICAN.ICANDM1RxSAF1.RedStopLampFlash_DIAG : KIBES_Signal/KIBES_Signal  MBDS_LibraryBlock=on  DatabaseKey=146  SignalName=ICAN.ICANDM1RxSAF1.RedStopLampFlash_DIAG  SymbolName=ICAN_ICANDM1RxSAF1_RedStopLampFlash_DIAG_000146  DataType=uint16  Init=1  Slope=1  Bias=0  DataSize=1  fpDataType=uint16  BlockIOType=Inport  DeviceType=0
  in_ICAN.ICANDM1RxSAF1.RedStopLamp_DIAG : KIBES_Signal/KIBES_Signal  MBDS_LibraryBlock=on  DatabaseKey=147  SignalName=ICAN.ICANDM1RxSAF1.RedStopLamp_DIAG  SymbolName=ICAN_ICANDM1RxSAF1_RedStopLamp_DIAG_000147  DataType=uint16  Init=1  Slope=1  Bias=0  DataSize=1  fpDataType=uint16  BlockIOType=Inport  DeviceType=0
  in_ICAN.ICANDM1RxSAF1.UndefinedActiveDtc : KIBES_Signal/KIBES_Signal  MBDS_LibraryBlock=on  DatabaseKey=402  SignalName=ICAN.ICANDM1RxSAF1.UndefinedActiveDtc  SymbolName=ICAN_ICANDM1RxSAF1_UndefinedActiveDtc_000402  DataType=boolean  Init=0  Slope=1  Bias=0  DataSize=1  fpDataType=boolean  BlockIOType=Inport  DeviceType=0
  in_ICANDM1RxSA19.GenericDTCFilter.SPN_1_FMI_1 : KIBES_Signal/KIBES_Signal  MBDS_LibraryBlock=on  DatabaseKey=157  SignalName=ICANDM1RxSA19.GenericDTCFilter.SPN_1_FMI_1  SymbolName=ICANDM1RxSA19_GenericDTCFilter_SPN_1_FMI_1_000157  DataType=boolean  Init=0  Slope=1  Bias=0  DataSize=1  fpDataType=boolean  BlockIOType=Inport  DeviceType=0
  in_ICANDM1RxSA19.GenericDTCFilter.SPN_5_FMI_10 : KIBES_Signal/KIBES_Signal  MBDS_LibraryBlock=on  DatabaseKey=158  SignalName=ICANDM1RxSA19.GenericDTCFilter.SPN_5_FMI_10  SymbolName=ICANDM1RxSA19_GenericDTCFilter_SPN_5_FMI_10_000158  DataType=boolean  Init=0  Slope=1  Bias=0  DataSize=1  fpDataType=boolean  BlockIOType=Inport  DeviceType=0
  in_ICANDM1RxSA19.GenericDTCFilter.SPN_6_FMI_1 : KIBES_Signal/KIBES_Signal  MBDS_LibraryBlock=on  DatabaseKey=159  SignalName=ICANDM1RxSA19.GenericDTCFilter.SPN_6_FMI_1  SymbolName=ICANDM1RxSA19_GenericDTCFilter_SPN_6_FMI_1_000159  DataType=boolean  Init=0  Slope=1  Bias=0  DataSize=1  fpDataType=boolean  BlockIOType=Inport  DeviceType=0
  in_IN_DigitalInputs.IN_DIG_01 : KIBES_Signal/KIBES_Signal  MBDS_LibraryBlock=on  DatabaseKey=73  SignalName=IN_DigitalInputs.IN_DIG_01  SymbolName=IN_DigitalInputs_IN_DIG_01_000073  DataType=boolean  Init=0  Slope=1  Bias=0  DataSize=1  fpDataType=boolean  BlockIOType=Inport  DeviceType=0
  in_IN_ICAN.IGenRx.I_Test1.MessageState : KIBES_Signal/KIBES_Signal  MBDS_LibraryBlock=on  DatabaseKey=90  SignalName=IN_ICAN.IGenRx.I_Test1.MessageState  SymbolName=IN_ICAN_IGenRx_I_Test1_MessageState_000090  DataType=uint16  Init=0  Slope=1  Bias=0  DataSize=1  fpDataType=uint16  BlockIOType=Inport  DeviceType=0
  in_IN_ICAN.IGenRx.I_Test1.Val_1 : KIBES_Signal/KIBES_Signal  MBDS_LibraryBlock=on  DatabaseKey=87  SignalName=IN_ICAN.IGenRx.I_Test1.Val_1  SymbolName=IN_ICAN_IGenRx_I_Test1_Val_1_000087  DataType=uint8  Init=0  Slope=1  Bias=0  DataSize=1  fpDataType=uint8  BlockIOType=Inport  DeviceType=0
  out_ICAN.ICANDM1RxSA19.MessageEnable : KIBES_Signal/KIBES_Signal  MBDS_LibraryBlock=on  DatabaseKey=154  SignalName=ICAN.ICANDM1RxSA19.MessageEnable  SymbolName=ICAN_ICANDM1RxSA19_MessageEnable_000154  DataType=boolean  Init=0  Slope=1  Bias=0  DataSize=1  fpDataType=boolean  BlockIOType=Outport  DeviceType=0
  out_ICAN.ICANDM1RxSAF1.MessageEnable : KIBES_Signal/KIBES_Signal  MBDS_LibraryBlock=on  DatabaseKey=138  SignalName=ICAN.ICANDM1RxSAF1.MessageEnable  SymbolName=ICAN_ICANDM1RxSAF1_MessageEnable_000138  DataType=boolean  Init=0  Slope=1  Bias=0  DataSize=1  fpDataType=boolean  BlockIOType=Outport  DeviceType=0
  out_OUT_ICAN.IGenRx.I_Test1.MessageEnable : KIBES_Signal/KIBES_Signal  MBDS_LibraryBlock=on  DatabaseKey=86  SignalName=OUT_ICAN.IGenRx.I_Test1.MessageEnable  SymbolName=OUT_ICAN_IGenRx_I_Test1_MessageEnable_000086  DataType=boolean  Init=0  Slope=1  Bias=0  DataSize=1  fpDataType=boolean  BlockIOType=Outport  DeviceType=0
  out_OUT_ICAN.IGenTx.I_Tes1.MessageEnable : KIBES_Signal/KIBES_Signal  MBDS_LibraryBlock=on  DatabaseKey=88  SignalName=OUT_ICAN.IGenTx.I_Tes1.MessageEnable  SymbolName=OUT_ICAN_IGenTx_I_Tes1_MessageEnable_000088  DataType=boolean  Init=0  Slope=1  Bias=0  DataSize=1  fpDataType=boolean  BlockIOType=Outport  DeviceType=0
  out_OUT_ICAN.IGenTx.I_Tes1.Val_1 : KIBES_Signal/KIBES_Signal  MBDS_LibraryBlock=on  DatabaseKey=89  SignalName=OUT_ICAN.IGenTx.I_Tes1.Val_1  SymbolName=OUT_ICAN_IGenTx_I_Tes1_Val_1_000089  DataType=uint8  Init=0  Slope=1  Bias=0  DataSize=1  fpDataType=uint8  BlockIOType=Outport  DeviceType=0
  wires:
  Constant3/1 -> out_OUT_ICAN.IGenTx.I_Tes1.Val_1/1
  Constant/1 -> out_OUT_ICAN.IGenRx.I_Test1.MessageEnable/1, out_OUT_ICAN.IGenTx.I_Tes1.MessageEnable/1, out_ICAN.ICANDM1RxSAF1.MessageEnable/1, out_ICAN.ICANDM1RxSA19.MessageEnable/1

== system MBDS_Applications/APP_MyApplicationT5 ==
  Constant1 : Constant  InitFcn=|  OutDataTypeStr=boolean
      | if(exist('MBDS_BlockCallback', 'file'))
      |    MBDS_BlockCallback('Update', gcb);  
      | end
  Constant3 : Constant  InitFcn=|  Value=2  OutDataTypeStr=uint8
      | if(exist('MBDS_BlockCallback', 'file'))
      |    MBDS_BlockCallback('Update', gcb);  
      | end
  in_IN_ACAN.TX_Gen.ACAN_TX_01.MessageState : KIBES_Signal/KIBES_Signal  MBDS_LibraryBlock=on  DatabaseKey=84  SignalName=IN_ACAN.TX_Gen.ACAN_TX_01.MessageState  SymbolName=IN_ACAN_TX_Gen_ACAN_TX_01_MessageState_000084  DataType=uint16  Init=0  Slope=1  Bias=0  DataSize=1  fpDataType=uint16  BlockIOType=Inport  DeviceType=0
  in_IN_DigitalInputs.IN_DIG_01 : KIBES_Signal/KIBES_Signal  MBDS_LibraryBlock=on  DatabaseKey=73  SignalName=IN_DigitalInputs.IN_DIG_01  SymbolName=IN_DigitalInputs_IN_DIG_01_000073  DataType=boolean  Init=0  Slope=1  Bias=0  DataSize=1  fpDataType=boolean  BlockIOType=Inport  DeviceType=0
  out_OUT_ACAN.TX_Gen.ACAN_TX_01.MessageEnable : KIBES_Signal/KIBES_Signal  MBDS_LibraryBlock=on  DatabaseKey=83  SignalName=OUT_ACAN.TX_Gen.ACAN_TX_01.MessageEnable  SymbolName=OUT_ACAN_TX_Gen_ACAN_TX_01_MessageEnable_000083  DataType=boolean  Init=0  Slope=1  Bias=0  DataSize=1  fpDataType=boolean  BlockIOType=Outport  DeviceType=0
  out_OUT_ACAN.TX_Gen.ACAN_TX_01.Val1 : KIBES_Signal/KIBES_Signal  MBDS_LibraryBlock=on  DatabaseKey=85  SignalName=OUT_ACAN.TX_Gen.ACAN_TX_01.Val1  SymbolName=OUT_ACAN_TX_Gen_ACAN_TX_01_Val1_000085  DataType=uint8  Init=0  Slope=1  Bias=0  DataSize=1  fpDataType=uint8  BlockIOType=Outport  DeviceType=0
  wires:
  Constant3/1 -> out_OUT_ACAN.TX_Gen.ACAN_TX_01.Val1/1
  Constant1/1 -> out_OUT_ACAN.TX_Gen.ACAN_TX_01.MessageEnable/1

== system MBDS_Applications/APP_MyApplicationT6 ==
  in_IN_DigitalInputs.IN_DIG_01 : KIBES_Signal/KIBES_Signal  MBDS_LibraryBlock=on  DatabaseKey=73  SignalName=IN_DigitalInputs.IN_DIG_01  SymbolName=IN_DigitalInputs_IN_DIG_01_000073  DataType=boolean  Init=0  Slope=1  Bias=0  DataSize=1  fpDataType=boolean  BlockIOType=Inport  DeviceType=0

== system MBDS_Applications/APP_MyApplication/AnalogIn ==

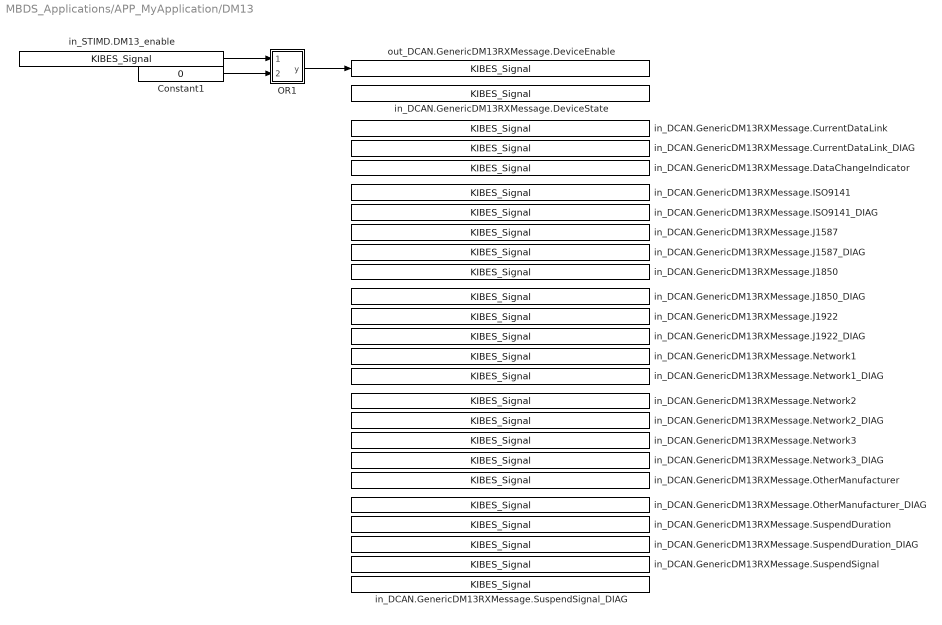
== system MBDS_Applications/APP_MyApplication/DM13 ==
  Constant1 : Constant  InitFcn=|  Value=0  OutDataTypeStr=boolean
      | if(exist('MBDS_BlockCallback', 'file'))
      |    MBDS_BlockCallback('Update', gcb);  
      | end
  OR1 : Subsystem  InitFcn=|  mask(OR){MBDS_LibraryBlock=on, BitwiseMode=off, Inputs=2, UseBitMask=off, BitMask='A1', OutDataTypeStr=Inherit: Inherit via back propagation, MBDS_BlockVersion=07.21.05}
      | if(exist('MBDS_BlockCallback', 'file'))
      |    MBDS_BlockCallback('Update', gcb);
      | end
      mask prompts: MBDS_LibraryBlock "MBDS library block"; BitwiseMode "Use 'bitwise' mode"; Inputs "Number of input ports:"; UseBitMask "Use bit mask"; BitMask "Bit mask:"; OutDataTypeStr "Output data type:"; MBDS_BlockVersion "Version:"
      mask help: Logical or bitwise OR operator. For multiple inputs, operators are applied across the inputs. For a single input, operators are applied across the input vector. In bitwise mode a bit mask can be applied onto single input signals.
      mask init: same as MBDS_Applications/APP_MyApplication/NOT
      mask Help: eval(['open([workdir(''library_dir:''),''\Blockset\help\'',get_param(gcb,''MaskType''),''.html''])'])
      mask Callback BitwiseMode:
      | if(exist('MBDS_BlockCallback', 'file'))
      |    MBDS_BlockCallback('BitwiseMode', gcb);
      | end
      mask Callback Inputs:
      | if(exist('MBDS_BlockCallback', 'file'))
      |    MBDS_BlockCallback('Inputs', gcb);
      | end
      mask Callback UseBitMask:
      | if(exist('MBDS_BlockCallback', 'file'))
      |    MBDS_BlockCallback('UseBitMask', gcb);
      | end
      mask Callback BitMask:
      | if(exist('MBDS_BlockCallback', 'file'))
      |    MBDS_BlockCallback('BitMask', gcb);
      | end
      mask TypeOptions OutDataTypeStr: Inherit: Inherit via back propagation | int8 | uint8 | int16 | uint16 | int32 | uint32 | boolean
      mask Callback OutDataTypeStr:
      | % Adopt Value
      | if(exist('MBDS_BlockCallback', 'file'))
      |    MBDS_BlockCallback('OutDataTypeStr', gcb);
      | end
      mask DialogControl ParameterTabVar0 Prompt: Main
      mask DialogControl ParameterTabVar01 Prompt: Signal Attributes
      mask DialogControl ParameterTabVar012 Prompt: Version
      mask Display:
      | % Show icon or block text
      | if(UseBitMask)
      |    if(isnumeric(BitMask))
      |       BitMaskString = ['0x',dec2hex(floor(BitMask))];
      |    elseif(ischar(BitMask))
      |       BitMaskString = ['0x',upper(BitMask)];
      |    else
      |       BitMaskString = '???';
      |    end
      |    disp(sprintf(['OR\n', BitMaskString]))
      | else
      |    disp('OR')
      | end
  in_DCAN.GenericDM13RXMessage.CurrentDataLink : KIBES_Signal/KIBES_Signal  MBDS_LibraryBlock=on  DatabaseKey=366  SignalName=DCAN.GenericDM13RXMessage.CurrentDataLink  SymbolName=DCAN_GenericDM13RXMessage_CurrentDataLink_000366  DataType=boolean  Init=0  Slope=1  Bias=0  DataSize=1  fpDataType=boolean  BlockIOType=Inport  DeviceType=0
  in_DCAN.GenericDM13RXMessage.CurrentDataLink_DIAG : KIBES_Signal/KIBES_Signal  MBDS_LibraryBlock=on  DatabaseKey=365  SignalName=DCAN.GenericDM13RXMessage.CurrentDataLink_DIAG  SymbolName=DCAN_GenericDM13RXMessage_CurrentDataLink_DIAG_000365  DataType=uint16  Init=1  Slope=1  Bias=0  DataSize=1  fpDataType=uint16  BlockIOType=Inport  DeviceType=0
  in_DCAN.GenericDM13RXMessage.DataChangeIndicator : KIBES_Signal/KIBES_Signal  MBDS_LibraryBlock=on  DatabaseKey=364  SignalName=DCAN.GenericDM13RXMessage.DataChangeIndicator  SymbolName=DCAN_GenericDM13RXMessage_DataChangeIndicator_000364  DataType=boolean  Init=0  Slope=1  Bias=0  DataSize=1  fpDataType=boolean  BlockIOType=Inport  DeviceType=0
  in_DCAN.GenericDM13RXMessage.DeviceState : KIBES_Signal/KIBES_Signal  MBDS_LibraryBlock=on  DatabaseKey=362  SignalName=DCAN.GenericDM13RXMessage.DeviceState  SymbolName=DCAN_GenericDM13RXMessage_DeviceState_000362  DataType=uint16  Init=0  Slope=1  Bias=0  DataSize=1  fpDataType=uint16  BlockIOType=Inport  DeviceType=0
  in_DCAN.GenericDM13RXMessage.ISO9141 : KIBES_Signal/KIBES_Signal  MBDS_LibraryBlock=on  DatabaseKey=361  SignalName=DCAN.GenericDM13RXMessage.ISO9141  SymbolName=DCAN_GenericDM13RXMessage_ISO9141_000361  DataType=boolean  Init=0  Slope=1  Bias=0  DataSize=1  fpDataType=boolean  BlockIOType=Inport  DeviceType=0
  in_DCAN.GenericDM13RXMessage.ISO9141_DIAG : KIBES_Signal/KIBES_Signal  MBDS_LibraryBlock=on  DatabaseKey=360  SignalName=DCAN.GenericDM13RXMessage.ISO9141_DIAG  SymbolName=DCAN_GenericDM13RXMessage_ISO9141_DIAG_000360  DataType=uint16  Init=1  Slope=1  Bias=0  DataSize=1  fpDataType=uint16  BlockIOType=Inport  DeviceType=0
  in_DCAN.GenericDM13RXMessage.J1587 : KIBES_Signal/KIBES_Signal  MBDS_LibraryBlock=on  DatabaseKey=359  SignalName=DCAN.GenericDM13RXMessage.J1587  SymbolName=DCAN_GenericDM13RXMessage_J1587_000359  DataType=boolean  Init=0  Slope=1  Bias=0  DataSize=1  fpDataType=boolean  BlockIOType=Inport  DeviceType=0
  in_DCAN.GenericDM13RXMessage.J1587_DIAG : KIBES_Signal/KIBES_Signal  MBDS_LibraryBlock=on  DatabaseKey=358  SignalName=DCAN.GenericDM13RXMessage.J1587_DIAG  SymbolName=DCAN_GenericDM13RXMessage_J1587_DIAG_000358  DataType=uint16  Init=1  Slope=1  Bias=0  DataSize=1  fpDataType=uint16  BlockIOType=Inport  DeviceType=0
  in_DCAN.GenericDM13RXMessage.J1850 : KIBES_Signal/KIBES_Signal  MBDS_LibraryBlock=on  DatabaseKey=357  SignalName=DCAN.GenericDM13RXMessage.J1850  SymbolName=DCAN_GenericDM13RXMessage_J1850_000357  DataType=boolean  Init=0  Slope=1  Bias=0  DataSize=1  fpDataType=boolean  BlockIOType=Inport  DeviceType=0
  in_DCAN.GenericDM13RXMessage.J1850_DIAG : KIBES_Signal/KIBES_Signal  MBDS_LibraryBlock=on  DatabaseKey=356  SignalName=DCAN.GenericDM13RXMessage.J1850_DIAG  SymbolName=DCAN_GenericDM13RXMessage_J1850_DIAG_000356  DataType=uint16  Init=1  Slope=1  Bias=0  DataSize=1  fpDataType=uint16  BlockIOType=Inport  DeviceType=0
  in_DCAN.GenericDM13RXMessage.J1922 : KIBES_Signal/KIBES_Signal  MBDS_LibraryBlock=on  DatabaseKey=355  SignalName=DCAN.GenericDM13RXMessage.J1922  SymbolName=DCAN_GenericDM13RXMessage_J1922_000355  DataType=boolean  Init=0  Slope=1  Bias=0  DataSize=1  fpDataType=boolean  BlockIOType=Inport  DeviceType=0
  in_DCAN.GenericDM13RXMessage.J1922_DIAG : KIBES_Signal/KIBES_Signal  MBDS_LibraryBlock=on  DatabaseKey=354  SignalName=DCAN.GenericDM13RXMessage.J1922_DIAG  SymbolName=DCAN_GenericDM13RXMessage_J1922_DIAG_000354  DataType=uint16  Init=1  Slope=1  Bias=0  DataSize=1  fpDataType=uint16  BlockIOType=Inport  DeviceType=0
  in_DCAN.GenericDM13RXMessage.Network1 : KIBES_Signal/KIBES_Signal  MBDS_LibraryBlock=on  DatabaseKey=353  SignalName=DCAN.GenericDM13RXMessage.Network1  SymbolName=DCAN_GenericDM13RXMessage_Network1_000353  DataType=boolean  Init=0  Slope=1  Bias=0  DataSize=1  fpDataType=boolean  BlockIOType=Inport  DeviceType=0
  in_DCAN.GenericDM13RXMessage.Network1_DIAG : KIBES_Signal/KIBES_Signal  MBDS_LibraryBlock=on  DatabaseKey=352  SignalName=DCAN.GenericDM13RXMessage.Network1_DIAG  SymbolName=DCAN_GenericDM13RXMessage_Network1_DIAG_000352  DataType=uint16  Init=1  Slope=1  Bias=0  DataSize=1  fpDataType=uint16  BlockIOType=Inport  DeviceType=0
  in_DCAN.GenericDM13RXMessage.Network2 : KIBES_Signal/KIBES_Signal  MBDS_LibraryBlock=on  DatabaseKey=351  SignalName=DCAN.GenericDM13RXMessage.Network2  SymbolName=DCAN_GenericDM13RXMessage_Network2_000351  DataType=boolean  Init=0  Slope=1  Bias=0  DataSize=1  fpDataType=boolean  BlockIOType=Inport  DeviceType=0
  in_DCAN.GenericDM13RXMessage.Network2_DIAG : KIBES_Signal/KIBES_Signal  MBDS_LibraryBlock=on  DatabaseKey=350  SignalName=DCAN.GenericDM13RXMessage.Network2_DIAG  SymbolName=DCAN_GenericDM13RXMessage_Network2_DIAG_000350  DataType=uint16  Init=1  Slope=1  Bias=0  DataSize=1  fpDataType=uint16  BlockIOType=Inport  DeviceType=0
  in_DCAN.GenericDM13RXMessage.Network3 : KIBES_Signal/KIBES_Signal  MBDS_LibraryBlock=on  DatabaseKey=349  SignalName=DCAN.GenericDM13RXMessage.Network3  SymbolName=DCAN_GenericDM13RXMessage_Network3_000349  DataType=boolean  Init=0  Slope=1  Bias=0  DataSize=1  fpDataType=boolean  BlockIOType=Inport  DeviceType=0
  in_DCAN.GenericDM13RXMessage.Network3_DIAG : KIBES_Signal/KIBES_Signal  MBDS_LibraryBlock=on  DatabaseKey=348  SignalName=DCAN.GenericDM13RXMessage.Network3_DIAG  SymbolName=DCAN_GenericDM13RXMessage_Network3_DIAG_000348  DataType=uint16  Init=1  Slope=1  Bias=0  DataSize=1  fpDataType=uint16  BlockIOType=Inport  DeviceType=0
  in_DCAN.GenericDM13RXMessage.OtherManufacturer : KIBES_Signal/KIBES_Signal  MBDS_LibraryBlock=on  DatabaseKey=347  SignalName=DCAN.GenericDM13RXMessage.OtherManufacturer  SymbolName=DCAN_GenericDM13RXMessage_OtherManufacturer_000347  DataType=boolean  Init=0  Slope=1  Bias=0  DataSize=1  fpDataType=boolean  BlockIOType=Inport  DeviceType=0
  in_DCAN.GenericDM13RXMessage.OtherManufacturer_DIAG : KIBES_Signal/KIBES_Signal  MBDS_LibraryBlock=on  DatabaseKey=346  SignalName=DCAN.GenericDM13RXMessage.OtherManufacturer_DIAG  SymbolName=DCAN_GenericDM13RXMessage_OtherManufacturer_DIAG_000346  DataType=uint16  Init=1  Slope=1  Bias=0  DataSize=1  fpDataType=uint16  BlockIOType=Inport  DeviceType=0
  in_DCAN.GenericDM13RXMessage.SuspendDuration : KIBES_Signal/KIBES_Signal  MBDS_LibraryBlock=on  DatabaseKey=345  SignalName=DCAN.GenericDM13RXMessage.SuspendDuration  SymbolName=DCAN_GenericDM13RXMessage_SuspendDuration_000345  DataType=uint16  Init=0  Slope=1  Bias=0  DataSize=1  fpDataType=uint16  BlockIOType=Inport  DeviceType=0
  in_DCAN.GenericDM13RXMessage.SuspendDuration_DIAG : KIBES_Signal/KIBES_Signal  MBDS_LibraryBlock=on  DatabaseKey=344  SignalName=DCAN.GenericDM13RXMessage.SuspendDuration_DIAG  SymbolName=DCAN_GenericDM13RXMessage_SuspendDuration_DIAG_000344  DataType=uint16  Init=1  Slope=1  Bias=0  DataSize=1  fpDataType=uint16  BlockIOType=Inport  DeviceType=0
  in_DCAN.GenericDM13RXMessage.SuspendSignal : KIBES_Signal/KIBES_Signal  MBDS_LibraryBlock=on  DatabaseKey=343  SignalName=DCAN.GenericDM13RXMessage.SuspendSignal  SymbolName=DCAN_GenericDM13RXMessage_SuspendSignal_000343  DataType=uint8  Init=0  Slope=1  Bias=0  DataSize=1  fpDataType=uint8  BlockIOType=Inport  DeviceType=0
  in_DCAN.GenericDM13RXMessage.SuspendSignal_DIAG : KIBES_Signal/KIBES_Signal  MBDS_LibraryBlock=on  DatabaseKey=342  SignalName=DCAN.GenericDM13RXMessage.SuspendSignal_DIAG  SymbolName=DCAN_GenericDM13RXMessage_SuspendSignal_DIAG_000342  DataType=uint16  Init=1  Slope=1  Bias=0  DataSize=1  fpDataType=uint16  BlockIOType=Inport  DeviceType=0
  in_STIMD.DM13_enable : KIBES_Signal/KIBES_Signal  MBDS_LibraryBlock=on  DatabaseKey=367  SignalName=STIMD.DM13_enable  SymbolName=STIMD_DM13_enable_000367  DataType=boolean  Init=0  Slope=1  Bias=0  DataSize=1  fpDataType=boolean  BlockIOType=Inport  DeviceType=2
  out_DCAN.GenericDM13RXMessage.DeviceEnable : KIBES_Signal/KIBES_Signal  MBDS_LibraryBlock=on  DatabaseKey=363  SignalName=DCAN.GenericDM13RXMessage.DeviceEnable  SymbolName=DCAN_GenericDM13RXMessage_DeviceEnable_000363  DataType=boolean  Init=0  Slope=1  Bias=0  DataSize=1  fpDataType=boolean  BlockIOType=Outport  DeviceType=0
  wires:
  in_STIMD.DM13_enable/1 -> OR1/1(u1)
  Constant1/1 -> OR1/2(u2)
  OR1/1(y) -> out_DCAN.GenericDM13RXMessage.DeviceEnable/1
